simulink model "airspeed_by_throttle_loop"  (R2014b)
settings: Solver=ode45  StartTime=0.0  StopTime=10.0  MaxStep=0.1  RelTol=1e-3
undefined symbols (not defined in the file or in its folder): a_V1, a_V2, k_i_V, k_p_V
settings Model: Creator=kunalmenda  LastModifiedBy=kunalmenda

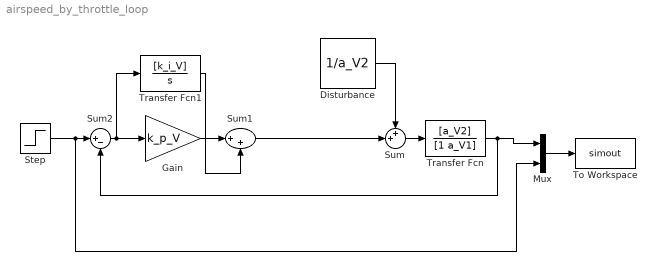
== system airspeed_by_throttle_loop ==
  Disturbance : Constant  Value=1/a_V2
  Gain : Gain  Gain=k_p_V
  Mux : Mux  Inputs=2
  Step : Step  After=10  SampleTime=0
  Sum : Sum  Inputs=++|
  Sum1 : Sum  Inputs=|++
  Sum2 : Sum  Inputs=|+-
  To Workspace : ToWorkspace  VariableName=simout  SaveFormat=Timeseries  SampleTime=-1
  Transfer Fcn : TransferFcn  Numerator=[a_V2]  Denominator=[1 a_V1]
  Transfer Fcn1 : TransferFcn  Numerator=[k_i_V]  Denominator=[1 0]
  wires:
  Sum2/1 -> Transfer Fcn1/1, Gain/1
  Step/1 -> Mux/2, Sum2/1
  Mux/1 -> To Workspace/1
  Gain/1 -> Sum1/1
  Transfer Fcn1/1 -> Sum1/2
  Sum1/1 -> Sum/2
  Disturbance/1 -> Sum/1
  Sum/1 -> Transfer Fcn/1
  Transfer Fcn/1 -> Sum2/2, Mux/1
